simulink model "aritmethic_demo"  (Simulink 6.3)
settings: Solver=ode45  StartTime=0.0  StopTime=10.0  RelTol=1e-3
settings Model: LastModifiedBy=Ms1

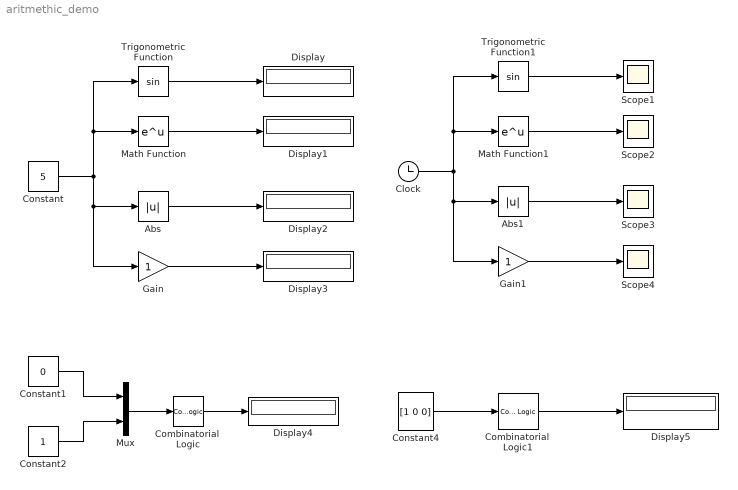
== system aritmethic_demo ==
  Abs : Abs  SaturateOnIntegerOverflow=on
  Abs1 : Abs  SaturateOnIntegerOverflow=on
  Clock : Clock
      settings: Decimation=10
  Combinatorial  Logic : CombinatorialLogic  TruthTable=[0;1;2;3]
  Combinatorial  Logic1 : CombinatorialLogic  TruthTable=[0;1;2;3;4;5;6;7]
  Constant : Constant  Value=5
  Constant1 : Constant  Value=0  OutDataTypeMode=boolean
  Constant2 : Constant  OutDataTypeMode=boolean
  Constant4 : Constant  Value=[1 0 0]  OutDataTypeMode=boolean
  Display{,1..5} (6 alike) : Display
  Gain : Gain  SaturateOnIntegerOverflow=on
  Gain1 : Gain  SaturateOnIntegerOverflow=on
  Math Function : Math  SaturateOnIntegerOverflow=on
  Math Function1 : Math  SaturateOnIntegerOverflow=on
  Mux : Mux  Inputs=2
  Scope{1..4} (4 alike) : Scope
      Scope2 settings: SaveName=ScopeData2
      Scope3 settings: SaveName=ScopeData3
      Scope4 settings: SaveName=ScopeData4
  Trigonometric Function : Trigonometry
  Trigonometric Function1 : Trigonometry
  wires:
  Constant/1 -> Trigonometric Function/1, Math Function/1, Abs/1, Gain/1
  Trigonometric Function/1 -> Display/1
  Math Function/1 -> Display1/1
  Abs/1 -> Display2/1
  Gain/1 -> Display3/1
  Clock/1 -> Trigonometric Function1/1, Math Function1/1, Abs1/1, Gain1/1
  Trigonometric Function1/1 -> Scope1/1
  Math Function1/1 -> Scope2/1
  Abs1/1 -> Scope3/1
  Gain1/1 -> Scope4/1
  Mux/1 -> Combinatorial  Logic/1
  Constant1/1 -> Mux/1
  Constant2/1 -> Mux/2
  Combinatorial  Logic/1 -> Display4/1
  Constant4/1 -> Combinatorial  Logic1/1
  Combinatorial  Logic1/1 -> Display5/1
